simulink model "datalogger"  (Simulink 7.5)
settings: Solver=ode45  StartTime=0.0  StopTime=10.0  RelTol=1e-3
undefined symbols (not defined in the file or in its folder): motohawk_get_faults
libraries: MotoHawk_lib x12
settings Model: Creator=Ethan  LastModifiedBy=Ethan

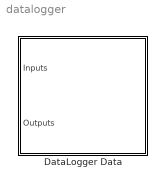
== system datalogger ==
  DataLogger Data : Subsystem

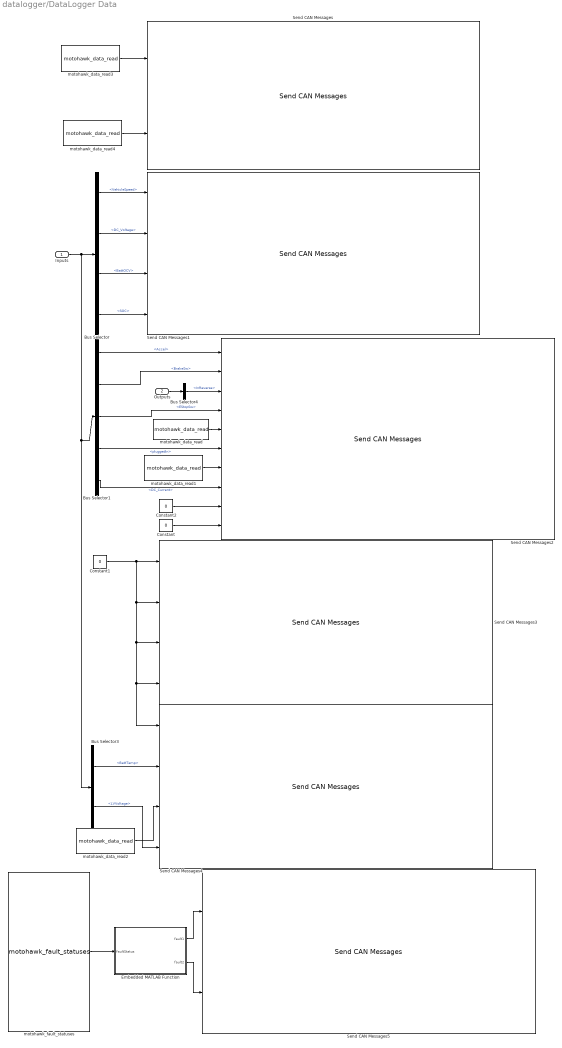
== system datalogger/DataLogger Data ==
  Inputs : Inport  OutDataType=sfix(16)  OutScaling=2^0
  Outputs : Inport  Port=2  OutDataType=sfix(16)  OutScaling=2^0
  Bus Selector : BusSelector  OutputSignals=Virtual.VehicleSpeed,Physical.DC_Voltage,Virtual.BattOCV,Virtual.SOC
  Bus Selector1 : BusSelector  OutputSignals=Physical.Accel,Physical.BrakeSw,Physical.EStopSw,Physical.NLG5.pluggedIn,Physical.DC_Current
  Bus Selector3 : BusSelector  OutputSignals=Physical.BattTemp,Physical.LVVoltage
  Bus Selector4 : BusSelector  OutputSignals=InReverse
  Constant : Constant  Value=0  OutDataType=sfix(16)  OutScaling=2^0
  Constant1 : Constant  Value=0  OutDataType=sfix(16)  OutScaling=2^0
  Constant2 : Constant  Value=0  OutDataType=sfix(16)  OutScaling=2^0
  Embedded MATLAB Function : Stateflow chart  TreatAsAtomicUnit=on
  Send CAN Messages : MotoHawk_lib/CAN Blocks/Send CAN Messages  bus=-2  nam='CAN_2'  msgl=ARDAQ_200  pace=5  labelwires=off
  Send CAN Messages1 : MotoHawk_lib/CAN Blocks/Send CAN Messages  bus=-2  nam='CAN_2'  msgl=ARDAQ_201  pace=5  labelwires=off
  Send CAN Messages2 : MotoHawk_lib/CAN Blocks/Send CAN Messages  bus=-2  nam='CAN_2'  msgl=ARDAQ_202  pace=5  labelwires=off
  Send CAN Messages3 : MotoHawk_lib/CAN Blocks/Send CAN Messages  bus=-2  nam='CAN_2'  msgl=ARDAQ_203  pace=5  labelwires=off
  Send CAN Messages4 : MotoHawk_lib/CAN Blocks/Send CAN Messages  bus=-2  nam='CAN_2'  msgl=ARDAQ_204  pace=5  labelwires=off
  Send CAN Messages5 : MotoHawk_lib/CAN Blocks/Send CAN Messages  bus=-2  nam='CAN_2'  msgl=ARDAQ_205  pace=5  labelwires=off
  motohawk_data_read : MotoHawk_lib/Data Storage Blocks/motohawk_data_read  source=Lookup By Name  structure=Scalar  operation=Read scalar from location by index  sz_vec=4  sz_row=2  sz_col=3  typ=uint8  nam='cCOn'  checkNull=on  struct_inst_name=''  struct_nam='MyStruct'
  motohawk_data_read1 : MotoHawk_lib/Data Storage Blocks/motohawk_data_read  source=Lookup By Name  structure=Scalar  operation=Read scalar from location by index  sz_vec=4  sz_row=2  sz_col=3  typ=uint8  nam='ChargingState'  checkNull=on  struct_inst_name=''  struct_nam='MyStruct'
  motohawk_data_read2 : MotoHawk_lib/Data Storage Blocks/motohawk_data_read  source=Lookup By Name  structure=Scalar  operation=Read scalar from location by index  sz_vec=4  sz_row=2  sz_col=3  typ=double  nam='cCSpeedSet'  checkNull=on  struct_inst_name=''  struct_nam='MyStruct'
  motohawk_data_read3 : MotoHawk_lib/Data Storage Blocks/motohawk_data_read  source=Lookup By Name  structure=Scalar  operation=Read scalar from location by index  sz_vec=4  sz_row=2  sz_col=3  typ=uint32  nam='startupCount'  checkNull=on  struct_inst_name=''  struct_nam='MyStruct'
  motohawk_data_read4 : MotoHawk_lib/Data Storage Blocks/motohawk_data_read  source=Lookup By Name  structure=Scalar  operation=Read scalar from location by index  sz_vec=4  sz_row=2  sz_col=3  typ=uint32  nam='totalOnTime'  checkNull=on  struct_inst_name=''  struct_nam='MyStruct'
  motohawk_fault_statuses : MotoHawk_lib/Fault Management Blocks/motohawk_fault_statuses  nam=motohawk_get_faults(bdroot)  status=Active
  wires:
  Inputs/1 -> Bus Selector/1, Bus Selector1/1, Bus Selector3/1
  Bus Selector/1 -> Send CAN Messages1/1  "<VehicleSpeed>"
  Bus Selector/2 -> Send CAN Messages1/2  "<DC_Voltage>"
  motohawk_data_read/1 -> Send CAN Messages2/5
  Bus Selector1/1 -> Send CAN Messages2/1  "<Accel>"
  Bus Selector1/2 -> Send CAN Messages2/2  "<BrakeSw>"
  Bus Selector1/3 -> Send CAN Messages2/4  "<EStopSw>"
  Bus Selector1/4 -> Send CAN Messages2/6  "<pluggedIn>"
  Bus Selector1/5 -> Send CAN Messages2/8  "<DC_Current>"
  motohawk_data_read1/1 -> Send CAN Messages2/7
  Constant1/1 -> Send CAN Messages3/1, Send CAN Messages3/2, Send CAN Messages3/3, Send CAN Messages3/4, Send CAN Messages4/1
  Bus Selector3/1 -> Send CAN Messages4/2  "<BattTemp>"
  Bus Selector3/2 -> Send CAN Messages4/4  "<LVVoltage>"
  motohawk_data_read2/1 -> Send CAN Messages4/3
  motohawk_fault_statuses/1 -> Embedded MATLAB Function/1(faultStatus)
  Embedded MATLAB Function/1(fault1) -> Send CAN Messages5/1
  Embedded MATLAB Function/2(fault2) -> Send CAN Messages5/2
  motohawk_data_read3/1 -> Send CAN Messages/1
  motohawk_data_read4/1 -> Send CAN Messages/2
  Outputs/1 -> Bus Selector4/1
  Bus Selector4/1 -> Send CAN Messages2/3  "<InReverse>"
  Bus Selector/3 -> Send CAN Messages1/3  "<BattOCV>"
  Bus Selector/4 -> Send CAN Messages1/4  "<SOC>"
  Constant/1 -> Send CAN Messages2/10
  Constant2/1 -> Send CAN Messages2/9

== matlab function DataLogger Data/Embedded MATLAB Function ==
  data: faultStatus input double; fault1 output double; fault2 output double
function [fault1,fault2] = fcn(faultStatus)
% This block supports the Embedded MATLAB subset.
% See the help menu for details. 
fault1 = uint32(0);
fault2 = uint32(0);
for i = 1:1:min(length(faultStatus), 32)
    fault1 = bitor(bitshift(fault1, 1), uint32(faultStatus(i)));
end
if length(faultStatus) <= 32
    fault1 = bitshift(fault1, 32 - length(faultStatus));
else
    for i = 33:1:min(length(faultStatus), 64)
        fault2 = bitor(bitshift(fault2, 1), uint32(faultStatus(i)));
    end
    fault2 = bitshift(fault2, 64 - length(faultStatus));
end
